simulink model "State_feedback"  (R2022a)
settings: Solver=VariableStepAuto  StartTime=0.0  StopTime=50  RelTol=1e-3
values from neighbouring files (symbols this model uses):
  A = [ 0 1 0 0; [-ks 0 ks 0]/ms;0 0 0 1;[ks 0 -ks-ku 0]/mu]    [H2.m]    (also in H2_alpha.m; H8_Alpha.m; H8_robust_mass.m = p*A1 + (1-p)*A2; Hinf.m)
  B = [0; Kc/ms; 0; -Kc/mu]    [H2.m]    (also in H2_alpha.m; H8_Alpha.m; H8_robust_mass.m = p*B1 + (1-p)*B2; Hinf.m)
  E = [0; 0; 0; ku/mu]    [H2.m]    (also in H2_alpha.m; H8_Alpha.m; H8_robust_mass.m = p*E1 + (1-p)*E2; Hinf.m)
  F = [Kc/ms;0;0;1]    [H2.m]    (also in H2_alpha.m; H8_Alpha.m; H8_robust_mass.m = p*F1 + (1-p)*F2; Hinf.m)
  H = [[-ks 0 ks 0]/ms;1 0 -1 0;0 0 1 0;0 0 0 0]    [H2.m]    (also in H2_alpha.m; H8_Alpha.m; H8_robust_mass.m = p*H1 + (1-p)*H2; Hinf.m)
  K = double(Y)*inv(double(X))    [H2.m]    (also in H2_alpha.m = double(Y)/(double(X)); H8_Alpha.m; H8_robust_f.m; H8_robust_mass.m)
  L = [0;0;-1;0]    [H2.m]    (also in H2_alpha.m; H8_Alpha.m; H8_robust_mass.m = p*L1 + (1-p)*L2; Hinf.m)
undefined symbols (not defined in the file or in its folder): Ad, Az, Bd, Bz, Cd, Cz, Dd, Dz
libraries: simulink x1
settings Model: Creator=User  LastModifiedBy=User

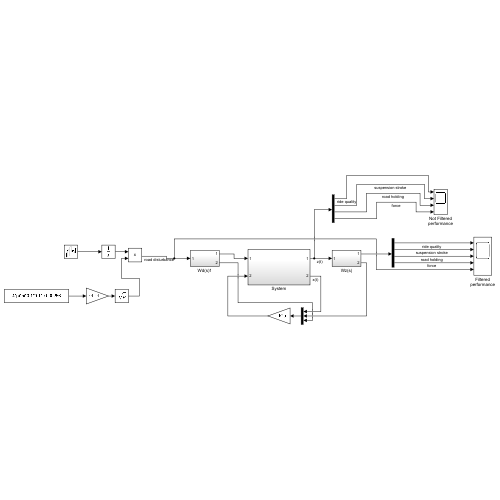
[thumbnail: Simulink's stored preview of the top-level diagram]
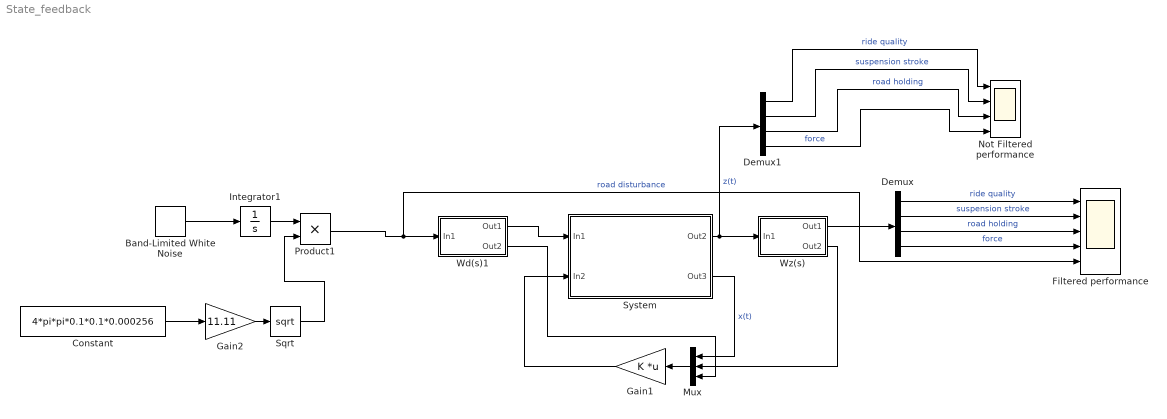
== system State_feedback ==
  Band-Limited White Noise : simulink/Sources/Band-Limited White Noise  Cov=[0.1]  Ts=0.1  seed=[23341]
  Constant : Constant  Value=4*pi*pi*0.1*0.1*0.000256
  Demux : Demux
  Demux1 : Demux
  Filtered performance : Scope  NumInputPorts=5
  Gain1 : Gain  Gain=K  Multiplication=Matrix(K*u)
  Gain2 : Gain  Gain=11.11
  Integrator1 : Integrator
  Mux : Mux  Inputs=3
  Not Filtered performance : Scope  NumInputPorts=4
  Product1 : Product
  Sqrt : Sqrt
  System : Subsystem
  Wd(s)1 : Subsystem
  Wz(s) : Subsystem
  wires:
  Wz(s)/2(Out2) -> Mux/2
  Wz(s)/1(Out1) -> Demux/1
  Demux/1 -> Filtered performance/1  "ride quality"
  System/1(Out2) -> Demux1/1, Wz(s)/1(In1)  "z(t)"
  Gain1/1 -> System/2(In2)
  Demux/2 -> Filtered performance/2  "suspension stroke"
  Mux/1 -> Gain1/1
  System/2(Out3) -> Mux/1  "x(t)"
  Wd(s)1/1(Out1) -> System/1(In1)
  Wd(s)1/2(Out2) -> Mux/3
  Demux/3 -> Filtered performance/3  "road holding"
  Demux1/1 -> Not Filtered performance/1  "ride quality"
  Demux1/2 -> Not Filtered performance/2  "suspension stroke"
  Demux1/3 -> Not Filtered performance/3  "road holding"
  Demux/4 -> Filtered performance/4  "force"
  Demux1/4 -> Not Filtered performance/4  "force"
  Integrator1/1 -> Product1/1
  Sqrt/1 -> Product1/2
  Band-Limited White Noise/1 -> Integrator1/1
  Gain2/1 -> Sqrt/1
  Constant/1 -> Gain2/1
  Product1/1 -> Filtered performance/5, Wd(s)1/1(In1)  "road disturbance"

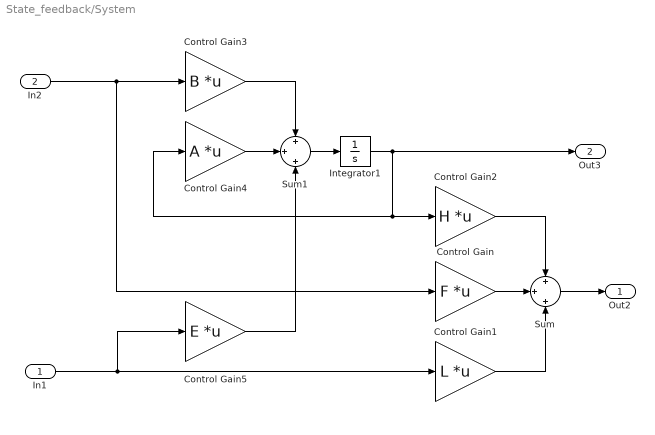
== system State_feedback/System ==
  In1 : Inport
  In2 : Inport  Port=2
  Control Gain : Gain  Gain=F  Multiplication=Matrix(K*u)
  Control Gain1 : Gain  Gain=L  Multiplication=Matrix(K*u)
  Control Gain2 : Gain  Gain=H  Multiplication=Matrix(K*u)
  Control Gain3 : Gain  Gain=B  Multiplication=Matrix(K*u)
  Control Gain4 : Gain  Gain=A  Multiplication=Matrix(K*u)
  Control Gain5 : Gain  Gain=E  Multiplication=Matrix(K*u)
  Integrator1 : Integrator
  Sum : Sum  Inputs=+|+|+
  Sum1 : Sum  Inputs=+|+|+
  Out2 : Outport
  Out3 : Outport  Port=2
  wires:
  Control Gain/1 -> Sum/2
  Control Gain2/1 -> Sum/1
  Control Gain1/1 -> Sum/3
  Control Gain3/1 -> Sum1/1
  Control Gain4/1 -> Sum1/2
  Sum1/1 -> Integrator1/1
  In2/1 -> Control Gain/1, Control Gain3/1
  In1/1 -> Control Gain5/1, Control Gain1/1
  Control Gain5/1 -> Sum1/3
  Integrator1/1 -> Out3/1, Control Gain4/1, Control Gain2/1
  Sum/1 -> Out2/1

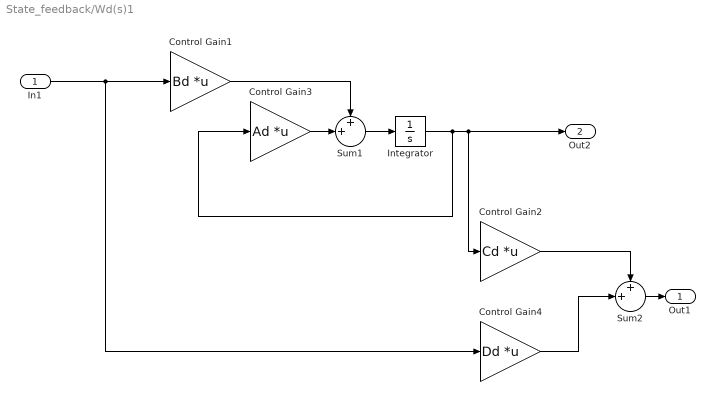
== system State_feedback/Wd(s)1 ==
  In1 : Inport
  Control Gain1 : Gain  Gain=Bd  Multiplication=Matrix(K*u)
  Control Gain2 : Gain  Gain=Cd  Multiplication=Matrix(K*u)
  Control Gain3 : Gain  Gain=Ad  Multiplication=Matrix(K*u)
  Control Gain4 : Gain  Gain=Dd  Multiplication=Matrix(K*u)
  Integrator : Integrator
  Sum1 : Sum  Inputs=++|
  Sum2 : Sum  Inputs=++|
  Out1 : Outport
  Out2 : Outport  Port=2
  wires:
  In1/1 -> Control Gain4/1, Control Gain1/1
  Integrator/1 -> Control Gain2/1, Out2/1, Control Gain3/1
  Sum1/1 -> Integrator/1
  Control Gain1/1 -> Sum1/1
  Control Gain3/1 -> Sum1/2
  Sum2/1 -> Out1/1
  Control Gain2/1 -> Sum2/1
  Control Gain4/1 -> Sum2/2

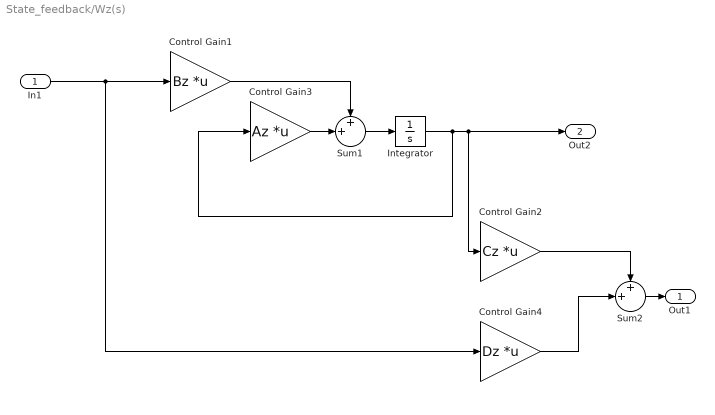
== system State_feedback/Wz(s) ==
  In1 : Inport
  Control Gain1 : Gain  Gain=Bz  Multiplication=Matrix(K*u)
  Control Gain2 : Gain  Gain=Cz  Multiplication=Matrix(K*u)
  Control Gain3 : Gain  Gain=Az  Multiplication=Matrix(K*u)
  Control Gain4 : Gain  Gain=Dz  Multiplication=Matrix(K*u)
  Integrator : Integrator
  Sum1 : Sum  Inputs=++|
  Sum2 : Sum  Inputs=++|
  Out1 : Outport
  Out2 : Outport  Port=2
  wires:
  In1/1 -> Control Gain4/1, Control Gain1/1
  Integrator/1 -> Control Gain2/1, Out2/1, Control Gain3/1
  Sum1/1 -> Integrator/1
  Control Gain1/1 -> Sum1/1
  Control Gain3/1 -> Sum1/2
  Sum2/1 -> Out1/1
  Control Gain2/1 -> Sum2/1
  Control Gain4/1 -> Sum2/2
